simulink model "delayTestVehicleModel"  (R2018b)
settings: Solver=FixedStepAuto  StartTime=0.0  StopTime=240  FixedStep=0.01  RelTol=1e-3
undefined symbols (not defined in the file or in its folder): Angular, Linear
libraries: robotlib x5, peGeneralControl x3, autolibshared x3, vehdynlibsteering x3, autolibutils x2, dspmathops x1, pe_lib x1, simulink x1
settings Model: Creator=ckreienk  LastModifiedBy=ckreienk

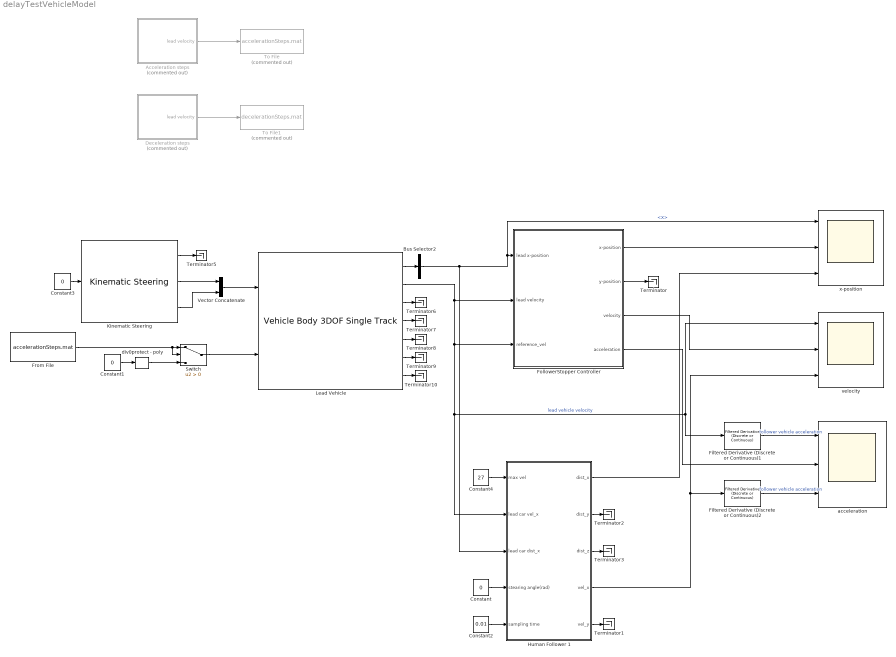
== system delayTestVehicleModel ==
  Acceleration steps : Subsystem  Commented=on
  Bus Selector2 : BusSelector  OutputSignals=InertFrm.Geom.Disp.X
  Constant : Constant  Value=0
  Constant1 : Constant  Value=0
  Constant2 : Constant  Value=0.01
  Constant3 : Constant  Value=0
  Constant4 : Constant  Value=27
  Deceleration steps : Subsystem  Commented=on
  Filtered Derivative (Discrete or Continuous)1 : peGeneralControl/Filtered Derivative (Discrete or Continuous)  K=1  T=0.1  B=20  A=-20  minRatio=10  Ts=-1
  Filtered Derivative (Discrete or Continuous)2 : peGeneralControl/Filtered Derivative (Discrete or Continuous)  K=1  T=0.1  B=20  A=-20  minRatio=10  Ts=-1
  FollowerStopper Controller : Subsystem
  From File : FromFile  FileName=accelerationSteps.mat  SampleTime=0.01
  Human Follower 1 : Subsystem
  Kinematic Steering : vehdynlibsteering/Kinematic Steering  StrgType=Ackerman  StrgRatioType=Constant  Loc=Front  NrmlFctr=0.01  TrckWdth=1  WhlBase=1.524  Db=0  StrgRng=1.25*pi  StrgAngBpts="[-6.2832   -5.0265   -3.7699   -2.5133   -1.2566         0    1.2566    2.5133    3.7699    5.0265    6.2832]"  StrgRatioTbl=|  StrgRatio=100  StrgArmLngth=0.1  RckCsLngth=0.5  TieRodLngth=0.248  D=0.2  PnnRadius=0.0057  PnnRadiusTbl="[0.0055    0.0055    0.0056    0.0057    0.0058    0.0057    0.0057    0.0057    0.0056    0.0055    0.0055]"  RodLngth=0.1  ParaArmLngth=0.9  aMode=2
      | [13.5000   13.3750   13.2500   13.1250   13.0000   13.0000   13.0000   13.1250   13.2500   13.3750   13.5000
      | ]
      settings: SourceProductName=Vehicle Dynamics Blockset
  Lead Vehicle : autolibshared/Vehicle Body 3DOF Single Track  trackMode=Dual  inputMode=External longitudinal velocity  frontSteerMode=on  rearSteerMode=off  windMode=off  muMode=off  extFMode=off  extMMode=off  aMode=2  NF=2  NR=2  m=2000  a=1.4  b=1.6  h=0.35  X_o=10  xdot_o=0  CalphaMode=off  sigmaMode=on  d=0  w=[1.4,1.4]  Cy_f=12e3  Cy_r=11e3  sigma_f=.1  sigma_r=.1  alpha_f_brk=[-.1 .1]  Cy_f_data=[-9e3 9e3]  alpha_r_brk=[-.1 .1]  Cy_r_data=[-9e3 9e3]  Y_o=0  ydot_o=0  Izz=4000  psi_o=0  r_o=0  Af=2  Cd=.3  Cl=.1  Cpm=.1  beta_w=[0:0.01:0.3]  Cs=[0:0.03:0.9]  Cym=[0:0.01:0.3]  Pabs=101325  Tair=273  g=9.81  mu=1  xdot_tol=.01  Fznom=5000  Fxtire_sat=7e4  Fytire_sat=7e4  longOff=0  latOff=0  vertOff=0
      settings: SourceProductName=Powertrain Blockset  SourceProductBaseCode=PW
  Switch : Switch  Criteria=u2 > Threshold
  Terminator{,1..3,5..10} (10 alike) : Terminator
  To File : ToFile  Commented=on  Filename=accelerationSteps.mat  SaveFormat=Timeseries
  To File1 : ToFile  Commented=on  Filename=decelerationSteps.mat  SaveFormat=Timeseries
  Vector Concatenate : Concatenate
  acceleration : Scope  NumInputPorts=3
  div0protect - poly : autolibutils/div0protect - poly  thresh=1e-3  aMode=2
      settings: SourceProductName=Powertrain Blockset  SourceProductBaseCode=PW
  velocity : Scope  NumInputPorts=3
  x-position : Scope  NumInputPorts=3
  wires:
  Vector Concatenate/1 -> Lead Vehicle/1
  Kinematic Steering/1 -> Terminator5/1
  Kinematic Steering/3 -> Vector Concatenate/2
  Lead Vehicle/6 -> Terminator9/1
  Lead Vehicle/2 -> FollowerStopper Controller/3(reference_vel), Filtered Derivative (Discrete or Continuous)1/1, velocity/1, Human Follower 1/2(lead car vel_x), FollowerStopper Controller/2(lead velocity)  "lead vehicle velocity"
  Kinematic Steering/2 -> Vector Concatenate/1
  Lead Vehicle/5 -> Terminator8/1
  Lead Vehicle/1 -> Bus Selector2/1
  Constant3/1 -> Kinematic Steering/1
  Lead Vehicle/7 -> Terminator10/1
  Lead Vehicle/3 -> Terminator6/1
  Lead Vehicle/4 -> Terminator7/1
  Bus Selector2/1 -> x-position/1, FollowerStopper Controller/1(lead x-position), Human Follower 1/3(lead car dist_x)  "<X>"
  FollowerStopper Controller/2(y-position) -> Terminator/1
  FollowerStopper Controller/1(x-position) -> x-position/2
  FollowerStopper Controller/3(velocity) -> velocity/2
  Filtered Derivative (Discrete or Continuous)1/1 -> acceleration/1  "follower vehicle acceleration"
  FollowerStopper Controller/4(acceleration) -> acceleration/2
  Constant1/1 -> div0protect - poly/1
  div0protect - poly/1 -> Switch/3
  Switch/1 -> Lead Vehicle/2
  Constant/1 -> Human Follower 1/4(stearing angle(rad))
  Constant2/1 -> Human Follower 1/5(sampling time)
  Human Follower 1/5(vel_y) -> Terminator1/1
  Human Follower 1/3(dist_z) -> Terminator3/1
  Human Follower 1/2(dist_y) -> Terminator2/1
  Human Follower 1/1(dist_x) -> x-position/3
  Human Follower 1/4(vel_x) -> velocity/3, Filtered Derivative (Discrete or Continuous)2/1
  Filtered Derivative (Discrete or Continuous)2/1 -> acceleration/3  "follower vehicle acceleration"
  Constant4/1 -> Human Follower 1/1(max vel)
  From File/1 -> Switch/2, Switch/1
  Acceleration steps/1(lead velocity) -> To File/1
  Deceleration steps/1(lead velocity) -> To File1/1

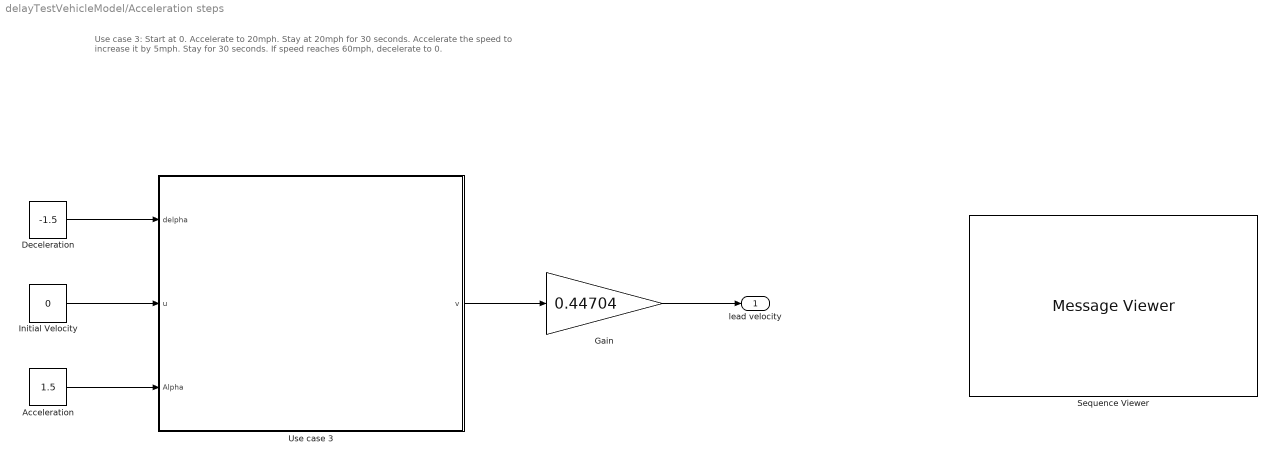
== system delayTestVehicleModel/Acceleration steps ==
  note: Use case 3:
      | Start at 0. Accelerate to 20mph. Stay at 20mph for 30 seconds.
      | Accelerate the speed to increase it by 5mph. Stay for 30 seconds.
      | If speed reaches 60mph, decelerate to 0.
  Acceleration : Constant  Value=1.5
  Deceleration : Constant  Value=-1.5
  Gain : Gain  Gain=0.44704
  Initial Velocity : Constant  Value=0
  Sequence Viewer : MessageViewer
  Use case 3 : Stateflow chart  TreatAsAtomicUnit=on
  lead velocity : Outport
  wires:
  Acceleration/1 -> Use case 3/3(Alpha)
  Initial Velocity/1 -> Use case 3/2(u)
  Deceleration/1 -> Use case 3/1(delpha)
  Use case 3/1(v) -> Gain/1
  Gain/1 -> lead velocity/1

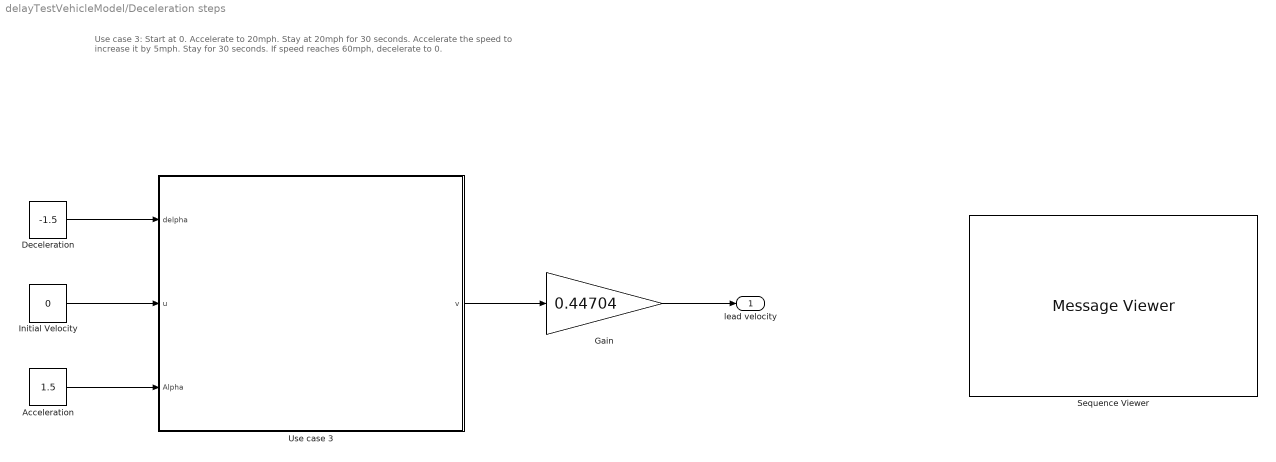
== system delayTestVehicleModel/Deceleration steps ==
  note: Use case 3:
      | Start at 0. Accelerate to 20mph. Stay at 20mph for 30 seconds.
      | Accelerate the speed to increase it by 5mph. Stay for 30 seconds.
      | If speed reaches 60mph, decelerate to 0.
  Acceleration : Constant  Value=1.5
  Deceleration : Constant  Value=-1.5
  Gain : Gain  Gain=0.44704
  Initial Velocity : Constant  Value=0
  Sequence Viewer : MessageViewer
  Use case 3 : Stateflow chart  TreatAsAtomicUnit=on
  lead velocity : Outport
  wires:
  Use case 3/1(v) -> Gain/1
  Deceleration/1 -> Use case 3/1(delpha)
  Initial Velocity/1 -> Use case 3/2(u)
  Acceleration/1 -> Use case 3/3(Alpha)
  Gain/1 -> lead velocity/1

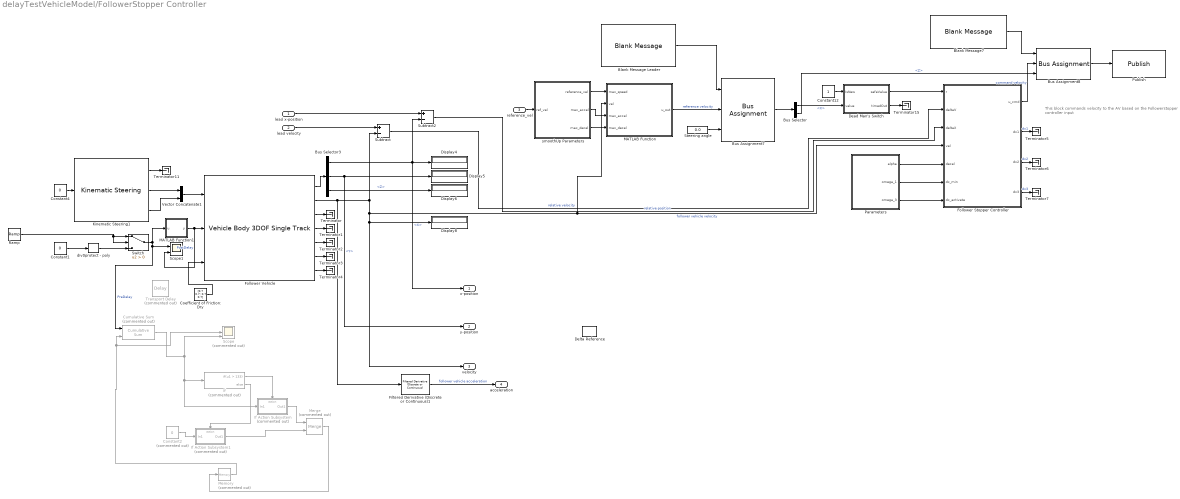
== system delayTestVehicleModel/FollowerStopper Controller ==
  note: This block commands velocity to the AV based
      | on the Followerstopper controller input
  lead x-position : Inport
  lead velocity : Inport  Port=2
  reference_vel : Inport  Port=3
  Blank Message Leader : robotlib/Blank Message  messageClass=Message  entityType=geometry_msgs/Twist  messageType=geometry_msgs/Twist  SampleTime=inf
      settings: SourceProductBaseCode=RO
  Blank Message7 : robotlib/Blank Message  messageClass=Message  entityType=geometry_msgs/Twist  messageType=geometry_msgs/Twist  SampleTime=inf
      settings: SourceProductBaseCode=RO
  Bus Assignment7 : BusAssignment  AssignedSignals=Linear.X,Angular.Z
  Bus Assignment8 : BusAssignment  AssignedSignals=Linear.X,Angular.Z
  Bus Selector : BusSelector  OutputSignals=Linear.X,Angular.Z
  Bus Selector3 : BusSelector  OutputSignals=InertFrm.Geom.Disp.X,InertFrm.Geom.Disp.Y,InertFrm.Geom.Disp.Z
  Coefficient of Friction: Dry : Constant  Value=[0.7 0.7; 0.7 0.7]
  Constant1 : Constant  Value=0
  Constant12 : Constant
  Constant2 : Constant  Commented=on  Value=0
  Constant4 : Constant  Value=0
  Cumulative Sum : dspmathops/Cumulative Sum  Commented=on  dim=Channels (running sum)  InputProcessing=Columns as channels (frame based)  reset_popup=Non-zero sample  roundingMode=Floor  overflowMode=off  outputDataTypeStr=Inherit: Same as accumulator  outputMin=[]  outputMax=[]  outputLastDataTypeStr=Inherit: Same as accumulator
      settings: SourceProductName=DSP System Toolbox
  Dead Man's Switch : Subsystem  TreatAsAtomicUnit=on  mask{stepSize=0.05, timeout=0.2}
      mask prompts: stepSize "Simulation step size"; timeout "Timeout (in seconds)"
      mask help: Interprets whether a new message has been recently received, and if so permits the data in 'value' to be passed through. Otherwise, 0 is outputted from 'safeValue'
      mask Help: Interprets whether a new message has been recently received, and if so permits the data in 'value' to be passed through. Otherwise, 0 is outputted from 'safeValue'
  Delta Reference : pe_lib/Connections/Delta Reference
      settings: SourceProductName=Simscape Power Systems  SourceProductBaseCode=PS
  Display{4..6,8} (4 alike) : Display
  Filtered Derivative (Discrete or Continuous)1 : peGeneralControl/Filtered Derivative (Discrete or Continuous)  K=1  T=0.1  B=20  A=-20  minRatio=10  Ts=-1
  Follower Stopper Controller : Subsystem
  Follower Vehicle : autolibshared/Vehicle Body 3DOF Single Track  trackMode=Dual  inputMode=External longitudinal velocity  frontSteerMode=on  rearSteerMode=off  windMode=off  muMode=on  extFMode=off  extMMode=off  aMode=2  NF=2  NR=2  m=2000  a=1.4  b=1.6  h=0.35  X_o=0  xdot_o=0  CalphaMode=off  sigmaMode=on  d=0  w=[1.4,1.4]  Cy_f=12e3  Cy_r=11e3  sigma_f=.1  sigma_r=.1  alpha_f_brk=[-.1 .1]  Cy_f_data=[-9e3 9e3]  alpha_r_brk=[-.1 .1]  Cy_r_data=[-9e3 9e3]  Y_o=0  ydot_o=0  Izz=4000  psi_o=0  r_o=0  Af=2  Cd=.3  Cl=.1  Cpm=.1  beta_w=[0:0.01:0.3]  Cs=[0:0.03:0.9]  Cym=[0:0.01:0.3]  Pabs=101325  Tair=273  g=9.81  mu=1  xdot_tol=.01  Fznom=5000  Fxtire_sat=7e4  Fytire_sat=7e4  longOff=0  latOff=0  vertOff=0
      settings: SourceProductName=Powertrain Blockset  SourceProductBaseCode=PW
  If : If  Commented=on  IfExpression=u1 > 133
  If Action Subsystem : Subsystem  Commented=on  TreatAsAtomicUnit=on
  If Action Subsystem1 : Subsystem  Commented=on  TreatAsAtomicUnit=on
  Kinematic Steering1 : vehdynlibsteering/Kinematic Steering  StrgType=Ackerman  StrgRatioType=Constant  Loc=Front  NrmlFctr=0.01  TrckWdth=1  WhlBase=1.524  Db=0  StrgRng=1.25*pi  StrgAngBpts="[-6.2832   -5.0265   -3.7699   -2.5133   -1.2566         0    1.2566    2.5133    3.7699    5.0265    6.2832]"  StrgRatioTbl=|  StrgRatio=100  StrgArmLngth=0.1  RckCsLngth=0.5  TieRodLngth=0.248  D=0.2  PnnRadius=0.0057  PnnRadiusTbl="[0.0055    0.0055    0.0056    0.0057    0.0058    0.0057    0.0057    0.0057    0.0056    0.0055    0.0055]"  RodLngth=0.1  ParaArmLngth=0.9  aMode=2
      | [13.5000   13.3750   13.2500   13.1250   13.0000   13.0000   13.0000   13.1250   13.2500   13.3750   13.5000
      | ]
      settings: SourceProductName=Vehicle Dynamics Blockset
  MATLAB Function : MATLAB Function  TreatAsAtomicUnit=on
  MATLAB Function1 : MATLAB Function  TreatAsAtomicUnit=on
  Memory : Memory  Commented=on
  Merge : Merge  Commented=on
  Parameters : Subsystem
  Publish : robotlib/Publish  topicSource=Specify your own  topic=cmd_vel  messageType=geometry_msgs/Twist  messageQueueLength=1
      settings: SourceProductBaseCode=RO
  Ramp : simulink/Sources/Ramp  slope=0.35  start=0  InitialOutput=3
  Scope : Scope  Commented=on  NumInputPorts=3
  Scope1 : Scope  NumInputPorts=2
  Steering angle : Constant  Value=0.0
  Subtract : Sum  Inputs=+-
  Subtract2 : Sum  Inputs=+-
  Switch : Switch  Criteria=u2 > Threshold
  Terminator{,1..7,11,15} (10 alike) : Terminator
  Transport Delay : TransportDelay  Commented=on  DelayTime=1.3
  Vector Concatenate1 : Concatenate
  div0protect - poly : autolibutils/div0protect - poly  thresh=1e-3  aMode=2
      settings: SourceProductName=Powertrain Blockset  SourceProductBaseCode=PW
  smoothUp Parameters : Subsystem
  x-position : Outport
  y-position : Outport  Port=2
  velocity : Outport  Port=3
  acceleration : Outport  Port=4
  wires:
  Follower Vehicle/7 -> Terminator4/1
  MATLAB Function/1(u_out) -> Bus Assignment7/2  "reference velocity"
  Constant4/1 -> Kinematic Steering1/1
  Parameters/3(omega_3) -> Follower Stopper Controller/7(dx_activate)
  Bus Selector3/2 -> y-position/1, Display5/1  "<Y>"
  Steering angle/1 -> Bus Assignment7/3
  Follower Vehicle/5 -> Terminator2/1
  Constant12/1 -> Dead Man's Switch/1(IsNew)
  Subtract2/1 -> Follower Stopper Controller/3(deltaX)  "relative position"
  Dead Man's Switch/1(safeValue) -> Follower Stopper Controller/1(r)
  Kinematic Steering1/1 -> Terminator11/1
  Bus Selector/1 -> Dead Man's Switch/2(value)  "<X>"
  Bus Selector3/3 -> Display6/1  "<Z>"
  Dead Man's Switch/2(timedOut) -> Terminator15/1
  Follower Vehicle/2 -> Filtered Derivative (Discrete or Continuous)1/1, velocity/1, Display8/1, MATLAB Function/2(vel), Follower Stopper Controller/4(vel), Subtract/2  "follower vehicle velocity"
  lead x-position/1 -> Subtract2/1
  Parameters/2(omega_1) -> Follower Stopper Controller/6(dx_min)
  Bus Selector3/1 -> x-position/1, Display4/1, Subtract2/2  "<X>"
  Vector Concatenate1/1 -> Follower Vehicle/1
  Subtract/1 -> Follower Stopper Controller/2(deltaV)  "relative velocity"
  Blank Message Leader/1 -> Bus Assignment7/1
  Filtered Derivative (Discrete or Continuous)1/1 -> acceleration/1  "follower vehicle acceleration"
  Bus Selector/2 -> Bus Assignment8/3  "<Z>"
  Bus Assignment8/1 -> Publish/1
  Bus Assignment7/1 -> Bus Selector/1
  smoothUp Parameters/1(reference_vel) -> MATLAB Function/1(max_speed)
  Coefficient of Friction: Dry/1 -> Follower Vehicle/3
  Follower Vehicle/6 -> Terminator3/1
  Blank Message7/1 -> Bus Assignment8/1
  smoothUp Parameters/2(max_accel) -> MATLAB Function/3(max_accel)
  Follower Vehicle/1 -> Bus Selector3/1
  Follower Vehicle/3 -> Terminator/1
  Kinematic Steering1/2 -> Vector Concatenate1/1
  Kinematic Steering1/3 -> Vector Concatenate1/2
  Parameters/1(alpha) -> Follower Stopper Controller/5(decel)
  lead velocity/1 -> Subtract/1
  smoothUp Parameters/3(max_decel) -> MATLAB Function/4(max_decel)
  Follower Vehicle/4 -> Terminator1/1
  Constant1/1 -> div0protect - poly/1
  div0protect - poly/1 -> Switch/3
  reference_vel/1 -> smoothUp Parameters/1(ref_vel)
  Follower Stopper Controller/1(u_cmd) -> Bus Assignment8/2  "command velocity"
  Follower Stopper Controller/2(dx1) -> Terminator5/1  "dx1"
  Follower Stopper Controller/3(dx2) -> Terminator6/1  "dx2"
  Follower Stopper Controller/4(dx3) -> Terminator7/1  "dx3"
  Cumulative Sum/1 -> Scope/3, If Action Subsystem/1(In1), If/1
  If/1 -> If Action Subsystem/Action
  If/2 -> If Action Subsystem1/Action
  Constant2/1 -> If Action Subsystem1/1(In1)
  If Action Subsystem/1(Out1) -> Merge/1
  If Action Subsystem1/1(Out1) -> Merge/2
  Merge/1 -> Memory/1
  Memory/1 -> Cumulative Sum/2, Scope/2
  MATLAB Function1/1(y) -> Scope1/2, Follower Vehicle/2  "PostDelay"
  Switch/1 -> MATLAB Function1/1(u), Cumulative Sum/1, Scope1/1  "PreDelay"
  Ramp/1 -> Switch/1, Switch/2

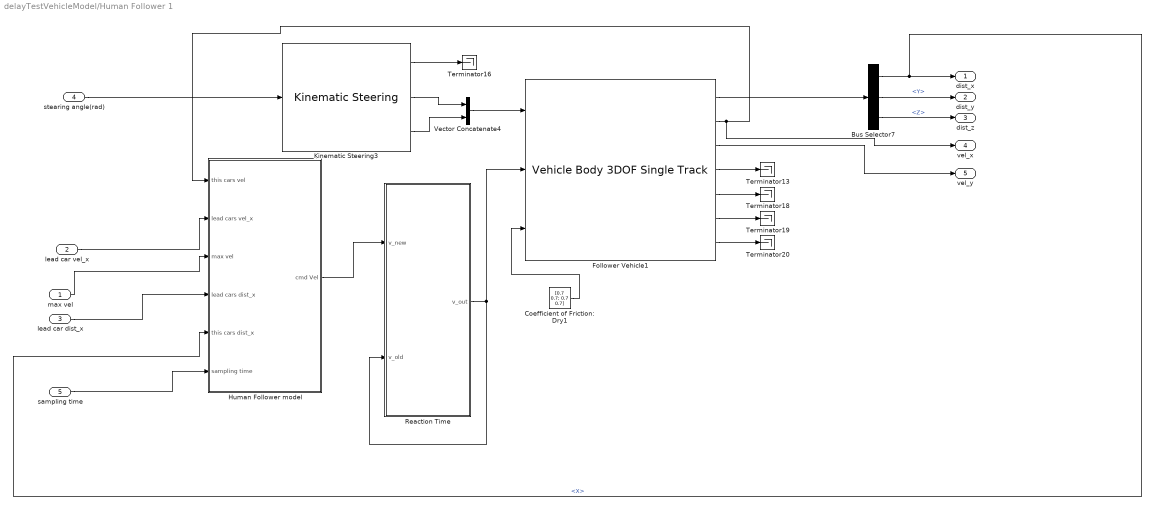
== system delayTestVehicleModel/Human Follower 1 ==
  max vel : Inport
  lead car vel_x : Inport  Port=2
  lead car dist_x : Inport  Port=3
  stearing angle(rad) : Inport  Port=4
  sampling time : Inport  Port=5
  Bus Selector7 : BusSelector  OutputSignals=InertFrm.Cg.Disp.X,InertFrm.Cg.Disp.Y,InertFrm.Cg.Disp.Z
  Coefficient of Friction: Dry1 : Constant  Value=[0.7 0.7; 0.7 0.7]
  Follower Vehicle1 : autolibshared/Vehicle Body 3DOF Single Track  trackMode=Dual  inputMode=External longitudinal velocity  frontSteerMode=on  rearSteerMode=off  windMode=off  muMode=on  extFMode=off  extMMode=off  aMode=2  NF=2  NR=2  m=2000  a=1.4  b=1.6  h=0.35  X_o=0  xdot_o=0  CalphaMode=off  sigmaMode=on  d=0  w=[1.4,1.4]  Cy_f=12e3  Cy_r=11e3  sigma_f=.1  sigma_r=.1  alpha_f_brk=[-.1 .1]  Cy_f_data=[-9e3 9e3]  alpha_r_brk=[-.1 .1]  Cy_r_data=[-9e3 9e3]  Y_o=0  ydot_o=0  Izz=4000  psi_o=0  r_o=0  Af=2  Cd=.3  Cl=.1  Cpm=.1  beta_w=[0:0.01:0.3]  Cs=[0:0.03:0.9]  Cym=[0:0.01:0.3]  Pabs=101325  Tair=273  g=9.81  mu=1  xdot_tol=.01  Fznom=5000  Fxtire_sat=7e4  Fytire_sat=7e4  longOff=0  latOff=0  vertOff=0
      settings: SourceProductName=Powertrain Blockset  SourceProductBaseCode=PW
  Human Follower model : Subsystem
  Kinematic Steering3 : vehdynlibsteering/Kinematic Steering  StrgType=Rack and pinion  StrgRatioType=Constant  Loc=Front  NrmlFctr=0.01  TrckWdth=1  WhlBase=1.524  Db=0  StrgRng=1.25*pi  StrgAngBpts="[-6.2832   -5.0265   -3.7699   -2.5133   -1.2566         0    1.2566    2.5133    3.7699    5.0265    6.2832]"  StrgRatioTbl=|  StrgRatio=100  StrgArmLngth=0.1  RckCsLngth=0.5  TieRodLngth=0.248  D=0.2  PnnRadius=0.0057  PnnRadiusTbl="[0.0055    0.0055    0.0056    0.0057    0.0058    0.0057    0.0057    0.0057    0.0056    0.0055    0.0055]"  RodLngth=0.1  ParaArmLngth=0.9  aMode=2
      | [13.5000   13.3750   13.2500   13.1250   13.0000   13.0000   13.0000   13.1250   13.2500   13.3750   13.5000
      | ]
      settings: SourceProductName=Vehicle Dynamics Blockset
  Reaction Time : Subsystem
  Terminator{13,16,18..20} (5 alike) : Terminator
  Vector Concatenate4 : Concatenate
  dist_x : Outport
  dist_y : Outport  Port=2
  dist_z : Outport  Port=3
  vel_x : Outport  Port=4
  vel_y : Outport  Port=5
  wires:
  Bus Selector7/3 -> dist_z/1  "<Z>"
  Follower Vehicle1/5 -> Terminator18/1
  max vel/1 -> Human Follower model/3(max vel)
  Follower Vehicle1/6 -> Terminator19/1
  Bus Selector7/1 -> dist_x/1, Human Follower model/5(this cars dist_x)  "<X>"
  Follower Vehicle1/4 -> Terminator13/1
  Follower Vehicle1/3 -> vel_y/1
  lead car vel_x/1 -> Human Follower model/2(lead cars vel_x)
  Follower Vehicle1/7 -> Terminator20/1
  Vector Concatenate4/1 -> Follower Vehicle1/1
  Follower Vehicle1/1 -> Bus Selector7/1
  Kinematic Steering3/1 -> Terminator16/1
  lead car dist_x/1 -> Human Follower model/4(lead cars dist_x)
  Bus Selector7/2 -> dist_y/1  "<Y>"
  Kinematic Steering3/2 -> Vector Concatenate4/1
  stearing angle(rad)/1 -> Kinematic Steering3/1
  Kinematic Steering3/3 -> Vector Concatenate4/2
  Follower Vehicle1/2 -> Human Follower model/1(this cars vel), vel_x/1
  Coefficient of Friction: Dry1/1 -> Follower Vehicle1/3
  sampling time/1 -> Human Follower model/6(sampling time)
  Reaction Time/1(v_out) -> Follower Vehicle1/2, Reaction Time/2(v_old)
  Human Follower model/1(cmd Vel) -> Reaction Time/1(v_new)

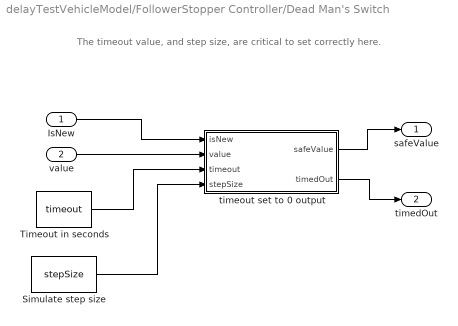
== system delayTestVehicleModel/FollowerStopper Controller/Dead Man's Switch ==
  note: The timeout value, and step size, are critical to set correctly here.
  IsNew : Inport
  value : Inport  Port=2
  Simulate step size : Constant  Value=stepSize
  Timeout in seconds : Constant  Value=timeout
  timeout set to 0 output : MATLAB Function  TreatAsAtomicUnit=on
  safeValue : Outport  InitialOutput=[0]
  timedOut : Outport  Port=2  InitialOutput=[0]
  wires:
  Simulate step size/1 -> timeout set to 0 output/4(stepSize)
  timeout set to 0 output/2(timedOut) -> timedOut/1
  Timeout in seconds/1 -> timeout set to 0 output/3(timeout)
  value/1 -> timeout set to 0 output/2(value)
  timeout set to 0 output/1(safeValue) -> safeValue/1
  IsNew/1 -> timeout set to 0 output/1(isNew)

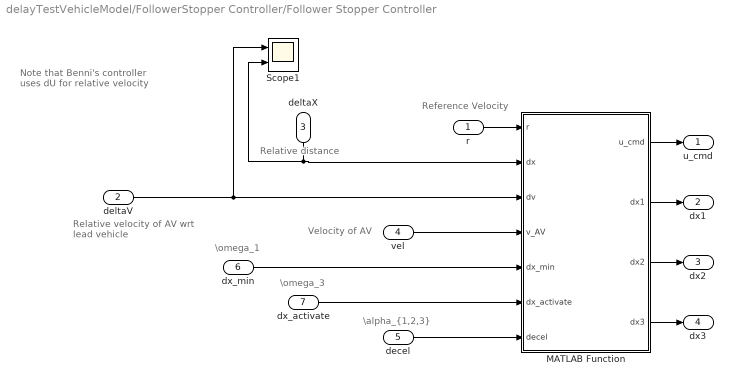
== system delayTestVehicleModel/FollowerStopper Controller/Follower Stopper Controller ==
  note: \alpha_{1,2,3}
  note: \omega_3
  note: \omega_1
  note: Relative distance
  note: Reference Velocity
  note: Velocity of AV
  note: Relative velocity of
      | AV wrt lead vehicle
  note: Note that Benni's
      | controller uses dU
      | for relative
      | velocity
  r : Inport
  deltaV : Inport  Port=2
  deltaX : Inport  Port=3
  vel : Inport  Port=4
  decel : Inport  Port=5
  dx_min : Inport  Port=6
  dx_activate : Inport  Port=7
  MATLAB Function : MATLAB Function  TreatAsAtomicUnit=on
  Scope1 : Scope  NumInputPorts=2
  u_cmd : Outport
  dx1 : Outport  Port=2
  dx2 : Outport  Port=3
  dx3 : Outport  Port=4
  wires:
  r/1 -> MATLAB Function/1(r)
  dx_activate/1 -> MATLAB Function/6(dx_activate)
  decel/1 -> MATLAB Function/7(decel)
  dx_min/1 -> MATLAB Function/5(dx_min)
  vel/1 -> MATLAB Function/4(v_AV)
  MATLAB Function/1(u_cmd) -> u_cmd/1
  deltaV/1 -> Scope1/1, MATLAB Function/3(dv)
  deltaX/1 -> Scope1/2, MATLAB Function/2(dx)
  MATLAB Function/2(dx1) -> dx1/1
  MATLAB Function/3(dx2) -> dx2/1
  MATLAB Function/4(dx3) -> dx3/1

== system delayTestVehicleModel/FollowerStopper Controller/If Action Subsystem ==
  In1 : Inport
  Action Port : ActionPort  ActionType=then
  Out1 : Outport
  wires:
  In1/1 -> Out1/1

== system delayTestVehicleModel/FollowerStopper Controller/If Action Subsystem1 ==
  In1 : Inport
  Action Port : ActionPort  ActionType=else
  Out1 : Outport
  wires:
  In1/1 -> Out1/1

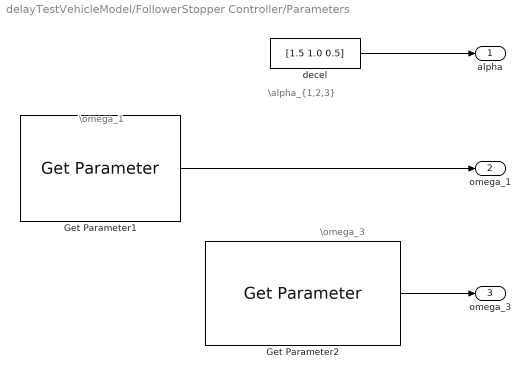
== system delayTestVehicleModel/FollowerStopper Controller/Parameters ==
  note: \alpha_{1,2,3}
  note: \omega_1
  note: \omega_3
  Get Parameter1 : robotlib/Get Parameter  ParameterSource=Specify your own  ParameterName=/dx_min  ParameterType=double  ParameterMaxArrayLength=16  ParameterInitialValue=4.5  SampleTime=-1  ShowErrorCodeOutput=off  ModelName=delayTestVehicleModel  BlockId=ParamGet_delayTestVehicleModel_52
      settings: SourceProductName=Robotics System Toolbox  SourceProductBaseCode=RO
  Get Parameter2 : robotlib/Get Parameter  ParameterSource=Specify your own  ParameterName=/dx_activate  ParameterType=double  ParameterMaxArrayLength=16  ParameterInitialValue=6.0  SampleTime=-1  ShowErrorCodeOutput=off  ModelName=delayTestVehicleModel  BlockId=ParamGet_delayTestVehicleModel_53
      settings: SourceProductName=Robotics System Toolbox  SourceProductBaseCode=RO
  decel : Constant  Value=[1.5 1.0 0.5]  OutDataTypeStr=double  SampleTime=-1
  alpha : Outport
  omega_1 : Outport  Port=2
  omega_3 : Outport  Port=3
  wires:
  decel/1 -> alpha/1
  Get Parameter1/1 -> omega_1/1
  Get Parameter2/1 -> omega_3/1

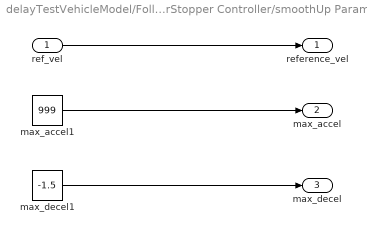
== system delayTestVehicleModel/FollowerStopper Controller/smoothUp Parameters ==
  ref_vel : Inport
  max_accel1 : Constant  Value=999
  max_decel1 : Constant  Value=-1.5
  reference_vel : Outport
  max_accel : Outport  Port=2
  max_decel : Outport  Port=3
  wires:
  ref_vel/1 -> reference_vel/1
  max_accel1/1 -> max_accel/1
  max_decel1/1 -> max_decel/1

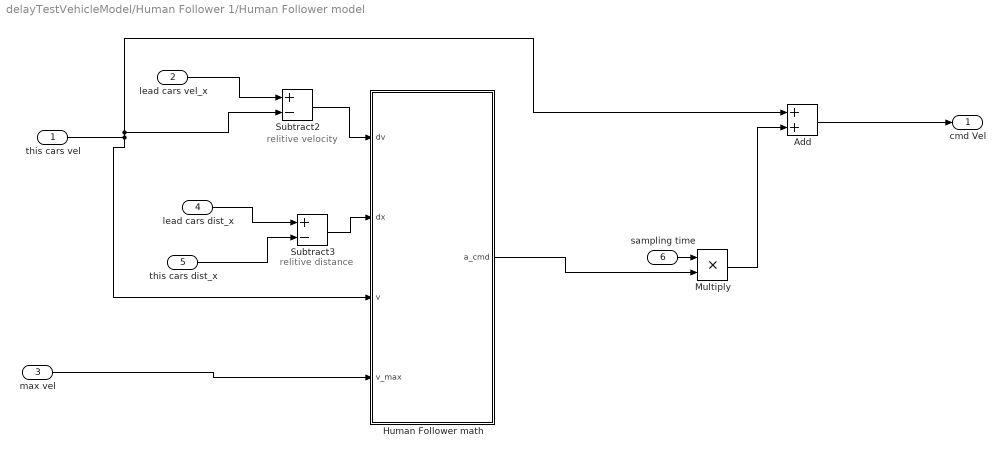
== system delayTestVehicleModel/Human Follower 1/Human Follower model ==
  note: relitive distance
  note: relitive velocity
  this cars vel : Inport
  lead cars vel_x : Inport  Port=2
  max vel : Inport  Port=3
  lead cars dist_x : Inport  Port=4
  this cars dist_x : Inport  Port=5
  sampling time : Inport  Port=6
  Add : Sum
  Human Follower math : Subsystem
  Multiply : Product
  Subtract2 : Sum  Inputs=+-
  Subtract3 : Sum  Inputs=+-
  cmd Vel : Outport
  wires:
  Add/1 -> cmd Vel/1
  lead cars dist_x/1 -> Subtract3/1
  this cars vel/1 -> Human Follower math/3(v), Add/1, Subtract2/2
  Human Follower math/1(a_cmd) -> Multiply/2
  Subtract3/1 -> Human Follower math/2(dx)
  Multiply/1 -> Add/2
  this cars dist_x/1 -> Subtract3/2
  Subtract2/1 -> Human Follower math/1(dv)
  max vel/1 -> Human Follower math/4(v_max)
  lead cars vel_x/1 -> Subtract2/1
  sampling time/1 -> Multiply/1

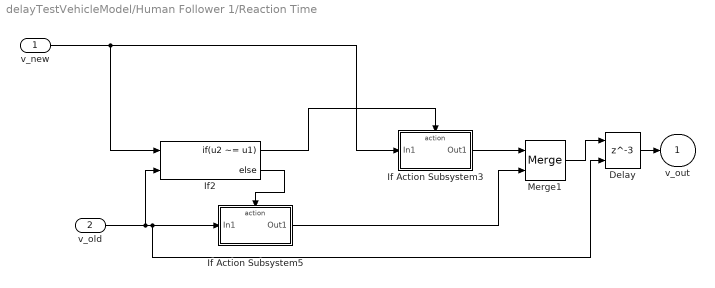
== system delayTestVehicleModel/Human Follower 1/Reaction Time ==
  v_new : Inport
  v_old : Inport  Port=2
  Delay : Delay  DelayLength=3  InitialConditionSource=Input port
      settings: InputPortMap=u0,p4
  If Action Subsystem3 : Subsystem  TreatAsAtomicUnit=on
  If Action Subsystem5 : Subsystem  TreatAsAtomicUnit=on
  If2 : If  NumInputs=2  IfExpression=u2 ~= u1
  Merge1 : Merge
  v_out : Outport
  wires:
  If Action Subsystem5/1(Out1) -> Merge1/2
  If2/1 -> If Action Subsystem3/Action
  If2/2 -> If Action Subsystem5/Action
  If Action Subsystem3/1(Out1) -> Merge1/1
  v_new/1 -> If2/1, If Action Subsystem3/1(In1)
  Merge1/1 -> Delay/1
  Delay/1 -> v_out/1
  v_old/1 -> If2/2, Delay/2, If Action Subsystem5/1(In1)

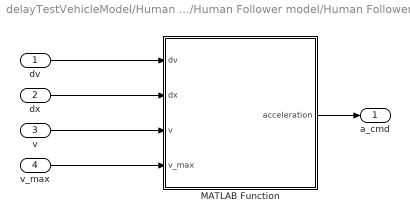
== system delayTestVehicleModel/Human Follower 1/Human Follower model/Human Follower math ==
  dv : Inport
  dx : Inport  Port=2
  v : Inport  Port=3
  v_max : Inport  Port=4
  MATLAB Function : MATLAB Function  TreatAsAtomicUnit=on
  a_cmd : Outport
  wires:
  v_max/1 -> MATLAB Function/4(v_max)
  MATLAB Function/1(acceleration) -> a_cmd/1
  v/1 -> MATLAB Function/3(v)
  dv/1 -> MATLAB Function/1(dv)
  dx/1 -> MATLAB Function/2(dx)

== system delayTestVehicleModel/Human Follower 1/Reaction Time/If Action Subsystem3 ==
  In1 : Inport
  Action Port : ActionPort  ActionType=then
  Out1 : Outport
  wires:
  In1/1 -> Out1/1

== system delayTestVehicleModel/Human Follower 1/Reaction Time/If Action Subsystem5 ==
  In1 : Inport
  Action Port : ActionPort  ActionType=else
  Out1 : Outport
  wires:
  In1/1 -> Out1/1

== matlab function delayTestVehicleModel/FollowerStopper Controller/Dead Man's Switch/timeout set to 0 output ==
  data: isNew input; safeValue output; value input; timeout input; timedOut output; stepSize input
function [safeValue,timedOut] = fcn(isNew,value,timeout,stepSize)
%#codegen
persistent sinceLastMsg
timedOut=true;
if isempty(sinceLastMsg)
    sinceLastMsg=(timeout/stepSize)+1;
end

safeValue=0;
% if no new message
% after timeout, we output 0
if( isNew == true )
    sinceLastMsg = 0;
else
    sinceLastMsg = sinceLastMsg+1;
end

% Note: we require step size as an input here, and depend on our
% system being executed at a regular rate, or bad things will happen
if( sinceLastMsg < timeout/stepSize )
    timedOut = false;
end
    
if( timedOut == false )
    safeValue = value;
end

== matlab function delayTestVehicleModel/FollowerStopper Controller/MATLAB Function ==
  settings: updateMethod=DISCRETE
  data: max_speed input; u_out output; vel input; max_accel input; max_decel input
function u_out = fcn(max_speed,vel,max_accel,max_decel)
% #codegen
persistent y

if isempty(y)
    y=vel;
end

dt=0.01;
if( y > max_speed + max_accel*dt)
    y = max(max_speed,y - abs(max_decel)*dt);
elseif( y < max_speed - abs(max_decel)*dt)
    y = min(max_speed,y + max_accel*dt);
else
    y = max_speed;
end

u_out = y;

== stateflow chart delayTestVehicleModel/Acceleration steps/Use case 3 ==
  note: Use case 3:
      | Start at 0. Accelerate to 20mph. Stay at 20mph for 30 seconds.
      | Accelerate the speed to increase it by 5mph. Stay for 30 seconds.
      | If speed reaches 60mph, decelerate to 0.
  state DecelerateTo0
    entry: entryState = nextState;
    during: v = getNewVaccel(v, delpha);
    exit: nextState = entryState + 1;
    note: STATE 3
  state zero
    entry: v = 0;
    during:v = 0;
    note: STATE 4
  state Accelerate
    entry: entryState = nextState; v = u2;
    during: v = getNewVaccel(v, Alpha);
    exit: nextState = entryState + 1;
    note: STATE 2
  state AccelerateTo60_init
    entry: entryState = 1; v = u;
    during: v = getNewVaccel(v, Alpha)
    exit:  nextState = entryState + 1;
    note: STATE 1
  state Hold
    entry: u2 = v;
    during: v = u2;
    exit:
    note: HOLD STATE
  DecelerateTo0 -> zero : [v <=0]
  Accelerate -> DecelerateTo0 [order 2] : [v > 35]
  Accelerate -> Hold [order 1] : [v - u2 >= 5 && v <= 35 ]
  Hold -> Accelerate : [after(30, sec)]
  (default) -> AccelerateTo60_init
  AccelerateTo60_init -> Hold : [v>=5 ]
  data: init_velocity function_input; acceleration function_input; new_vel function_output; delpha input; u input; Alpha input; v output =0; u2 local =0; entryState local =0; nextState local =0
  function new_vel = getNewVaccel(init_velocity, acceleration):
    | function new_vel = getNewVaccel(init_velocity, acceleration)
    | 
    | new_vel = init_velocity + (acceleration*0.05);
    | 
    | end

== stateflow chart delayTestVehicleModel/Deceleration steps/Use case 3 ==
  note: Use case 3:
      | Start at 0. Accelerate to 20mph. Stay at 20mph for 30 seconds.
      | Accelerate the speed to increase it by 5mph. Stay for 30 seconds.
      | If speed reaches 60mph, decelerate to 0.
  state DecelerateTo0
    entry: entryState = nextState;
    during: v = getNewVdecel(v, delpha);
    exit: nextState = entryState + 1;
    note: STATE 3
  state zero
    entry: v = 0;
    during:v = 0;
    note: STATE 4
  state Accelerate
    entry: entryState = nextState; v = u2;
    during: v = getNewVdecel(v, Alpha);
    exit: nextState = entryState + 1;
    note: STATE 2
  state AccelerateTo60_init
    entry: entryState = 1; v = u;
    during: v = getNewVaccel(v, Alpha)
    exit:  nextState = entryState + 1;
    note: STATE 1
  state Hold
    entry: u2 = v;
    during: v = u2;
    exit:
    note: HOLD STATE
  DecelerateTo0 -> zero : [v <=0]
  Accelerate -> DecelerateTo0 [order 2] : [v < 5]
  Accelerate -> Hold [order 1] : [u2 - v >= 5 && v >= 5 ]
  Hold -> Accelerate : [after(30, sec)]
  (default) -> AccelerateTo60_init
  AccelerateTo60_init -> Hold : [v>=35 ]
  data: init_velocity function_input; deceleration function_input; new_vel function_output; init_velocity function_input; acceleration function_input; new_vel function_output; delpha input; u input; Alpha input; v output =0; u2 local =0; entryState local =0; nextState local =0
  function new_vel = getNewVdecel(init_velocity, deceleration):
    | function new_vel = getNewVdecel(init_velocity, deceleration)
    | 
    | new_vel = init_velocity - abs(deceleration*0.05);
    | 
    | end
  function new_vel = getNewVaccel(init_velocity, acceleration):
    | function new_vel = getNewVaccel(init_velocity, acceleration)
    | 
    | new_vel = init_velocity + (acceleration*0.05);
    | 
    | end

== matlab function delayTestVehicleModel/Human Follower 1/Human Follower model/Human Follower math/MATLAB Function ==
  data: dv input; dx input; v input; v_max input; acceleration output
function acceleration = fcn(dv, dx, v, v_max)
sd = 2;

if v + dv < 0
    V = 0;
end
if dx <= sd
    V = 0;
elseif dx <= 35
    V = dx - (5 + sd);
else
    V = 30;
end

if dv + v <= v_max
    w = v + dv;
else
    w = v_max;
end

acceleration = 0.1*(V-v) + 0.5*(w-v);

== matlab function delayTestVehicleModel/FollowerStopper Controller/Follower Stopper Controller/MATLAB Function ==
  data: r input; u_cmd output; dx input; dv input; v_AV input; dx_min input; dx_activate input; decel input; dx1 output; dx2 output; dx3 output
function [u_cmd,dx1,dx2,dx3] = fcn(r,dx,dv,v_AV,...
    dx_min,dx_activate,decel)
%#codegen
% Safety controller, based on quadratic bands.
% Input: r = desired velocity (from other models)
%          dx = estimate of gap to vehicle ahead
%          dv = estimate of time derivative of dx (= velocity difference)
%         v_AV = velocity of AV
%      dx_min = minimum distance
% dx_activate = distance below which controller does something
%       decel = vector of three deceleration values for parabolas
% Out:  u_cmd = actual velocity commanded (always u_cmd<=U)
%
% Controller-specific parameters
dx_mid = (dx_min+dx_activate)/2; % mid distance, where v_lead is commanded
% Lead vehicle velocity
v_lead = v_AV+dv; % velocity of lead vehicle
v_lead = max(v_lead,0); % lead vehicle cannot go backwards
v = min(r,v_lead); % safety velocity cannot exceed desired velocity U
% Treatment of positive dv-values
dv = min(dv,0); % domains for dv>0 same as dv=0
% For given dv, dx-values of band boundaries
dx1 = dx_min+1/(2*decel(1))*dv.^2;
dx2 = dx_mid+1/(2*decel(2))*dv.^2;
dx3 = dx_activate+1/(2*decel(3))*dv.^2;

% Actual commanded velocity
dt = 0.01;
max_accel = 1.5;
smoothChange = v_AV + max_accel*dt;
u_cmd = double((dx<=dx1).*(0)+...
    (dx1<dx&dx<=dx2).*(min(v*(dx-dx1)/(dx2-dx1) , smoothChange))+...
    (dx2<dx&dx<=dx3).*(min(v + (r-v)*(dx-dx2)/(dx3-dx2) , smoothChange))+...
    (dx3<dx).*(min(r , smoothChange)));

== matlab function delayTestVehicleModel/FollowerStopper Controller/MATLAB Function1 ==
  settings: updateMethod=DISCRETE
  data: u input; y output
function y = Delay_200(u)
persistent bf
if isempty(bf)
   bf = zeros(1,200);
end

bf(2:end) = bf(1:end -1);
bf(1) = u;
y= bf(end);
